simulink model "AdaptiveCruiseControl"  (R2015a)
settings: Solver=ode45  StartTime=0.0  StopTime=250  RelTol=3e-14
libraries: simulink x2
settings Model: CovSFcnEnable=off  Creator=chizom  LastModifiedBy=WORNU CHIZOM

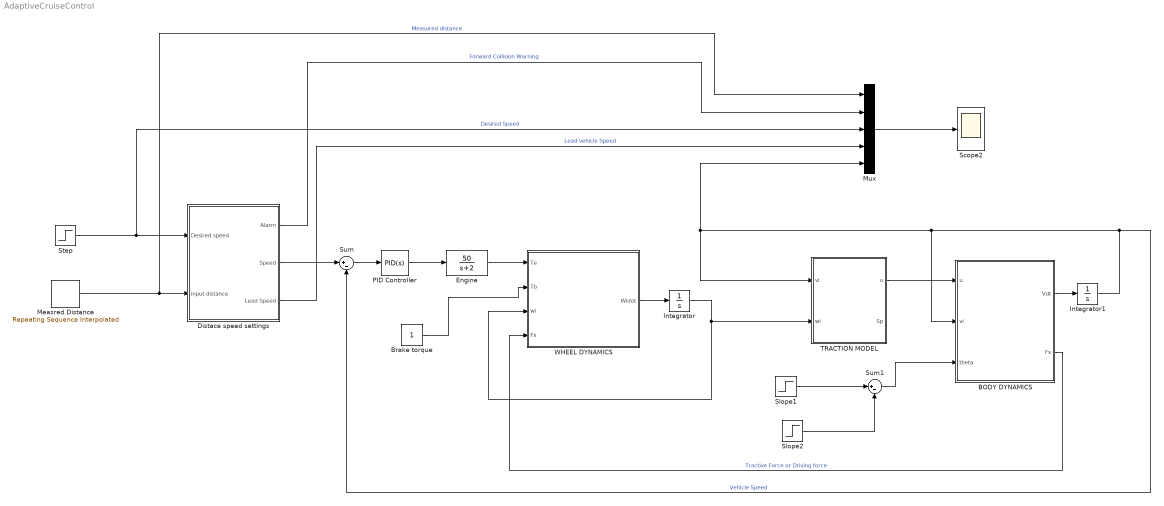
== system AdaptiveCruiseControl ==
  BODY DYNAMICS : Subsystem
  Brake torque : Constant
  Distace speed settings : Subsystem
  Engine : TransferFcn  Numerator=[50]  Denominator=[1 2]
  Integrator : Integrator
  Integrator1 : Integrator  InitialCondition=1
  Measred Distance : simulink/Sources/Repeating Sequence Interpolated  OutValues=[40 30 20 10 8 7 6 6 6 6 6 6].'  TimeValues=[20 40 60 80 100 120 140 160 180 200 220 240].'  LookUpMeth=Interpolation-Use End Values  tsamp=0.001  OutMin=[]  OutMax=[]  OutDataTypeStr=Inherit: Inherit via back propagation  OutDataType=fixdt(0,8)  OutScaling=2^-10
  Mux : Mux  Inputs=5
  PID Controller : simulink/Continuous/PID Controller  Controller=PID  TimeDomain=Continuous-time  SampleTime=-1  IntegratorMethod=Forward Euler  FilterMethod=Forward Euler  Form=Parallel  UseFilter=on  ControllerParametersSource=internal  P=20.88  I=20.88  D=13.92  N=1  InitialConditionSource=internal  InitialConditionForIntegrator=0  InitialConditionForFilter=0  ExternalReset=none  LimitOutput=off  UpperSaturationLimit=inf  LowerSaturationLimit=-inf  LinearizeAsGain=on  AntiWindupMode=none  Kb=1  TrackingMode=off  Kt=1  PParamMin=[]  PParamMax=[]  IParamMin=[]  IParamMax=[]  DParamMin=[]  DParamMax=[]  NParamMin=[]  NParamMax=[]  KbParamMin=[]  KbParamMax=[]  KtParamMin=[]  KtParamMax=[]  POutMin=[]  POutMax=[]  IOutMin=[]  IOutMax=[]  DOutMin=[]  DOutMax=[]  NOutMin=[]  NOutMax=[]  KbOutMin=[]  KbOutMax=[]  KtOutMin=[]  KtOutMax=[]  IntegratorOutMin=[]  IntegratorOutMax=[]  FilterOutMin=[]  FilterOutMax=[]  SumOutMin=[]  SumOutMax=[]  SumI1OutMin=[]  SumI1OutMax=[]  SumI2OutMin=[]  SumI2OutMax=[]  SumI3OutMin=[]  SumI3OutMax=[]  SumDOutMin=[]  SumDOutMax=[]  SaturationOutMin=[]  SaturationOutMax=[]  IntegratorContinuousStateAttributes=''  IntegratorStateMustResolveToSignalObject=off  IntegratorRTWStateStorageClass=Auto  FilterContinuousStateAttributes=''  FilterStateMustResolveToSignalObject=off  FilterRTWStateStorageClass=Auto  DifferentiatorICPrevScaledInput=0  DifferentiatorOutMin=[]  DifferentiatorOutMax=[]
  Scope2 : Scope
      settings: TickLabels=on  ShowLegends=on  TimeRange=250  YMin=0  YMax=70
  Slope1 : Step  Time=100  After=0  SampleTime=0
  Slope2 : Step  Time=200  After=0  SampleTime=0
  Step : Step  Time=0  Before=0.0001  After=30  SampleTime=0
  Sum : Sum  Inputs=|+-
  Sum1 : Sum  Inputs=|+-
  TRACTION MODEL : Subsystem
  WHEEL DYNAMICS : Subsystem
  wires:
  Integrator/1 -> WHEEL DYNAMICS/3(wi), TRACTION MODEL/2(wi)
  WHEEL DYNAMICS/1(Widot) -> Integrator/1
  Engine/1 -> WHEEL DYNAMICS/1(Te)
  TRACTION MODEL/1(u) -> BODY DYNAMICS/1(u)
  BODY DYNAMICS/1(Vdt) -> Integrator1/1
  Integrator1/1 -> TRACTION MODEL/1(vi), Mux/5, BODY DYNAMICS/2(vi), Sum/2  "Vehicle Speed"
  Distace speed settings/2(Speed) -> Sum/1
  Mux/1 -> Scope2/1
  Step/1 -> Mux/3, Distace speed settings/1(Desired speed)  "Desired Speed"
  Measred Distance/1 -> Mux/1, Distace speed settings/2(input distance)  "Measured distance"
  Sum1/1 -> BODY DYNAMICS/3(theta)
  Slope1/1 -> Sum1/1
  Slope2/1 -> Sum1/2
  Sum/1 -> PID Controller/1
  PID Controller/1 -> Engine/1
  Distace speed settings/1(Alarm) -> Mux/2  "Forward Collision Warning"
  Distace speed settings/3(Lead Speed) -> Mux/4  "Lead vehicle Speed"
  BODY DYNAMICS/2(Fx) -> WHEEL DYNAMICS/4(Fx)  "Tractive Force or Driving force"
  Brake torque/1 -> WHEEL DYNAMICS/2(Tb)

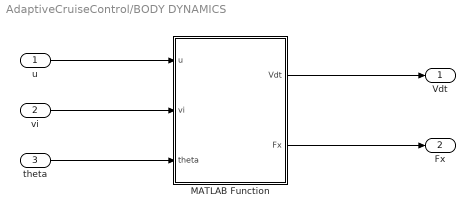
== system AdaptiveCruiseControl/BODY DYNAMICS ==
  u : Inport
  vi : Inport  Port=2
  theta : Inport  Port=3
  MATLAB Function : MATLAB Function  TreatAsAtomicUnit=on
  Vdt : Outport
  Fx : Outport  Port=2
  wires:
  MATLAB Function/1(Vdt) -> Vdt/1
  vi/1 -> MATLAB Function/2(vi)
  theta/1 -> MATLAB Function/3(theta)
  u/1 -> MATLAB Function/1(u)
  MATLAB Function/2(Fx) -> Fx/1

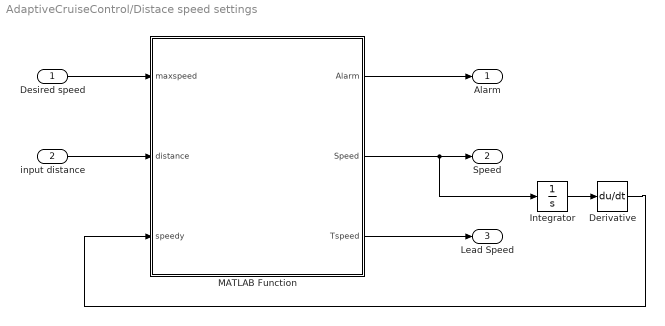
== system AdaptiveCruiseControl/Distace speed settings ==
  Desired speed : Inport
  input distance : Inport  Port=2
  Derivative : Derivative
  Integrator : Integrator
  MATLAB Function : MATLAB Function  TreatAsAtomicUnit=on
  Alarm : Outport
  Speed : Outport  Port=2
  Lead Speed : Outport  Port=3
  wires:
  MATLAB Function/1(Alarm) -> Alarm/1
  Desired speed/1 -> MATLAB Function/1(maxspeed)
  input distance/1 -> MATLAB Function/2(distance)
  MATLAB Function/3(Tspeed) -> Lead Speed/1
  MATLAB Function/2(Speed) -> Integrator/1, Speed/1
  Integrator/1 -> Derivative/1
  Derivative/1 -> MATLAB Function/3(speedy)

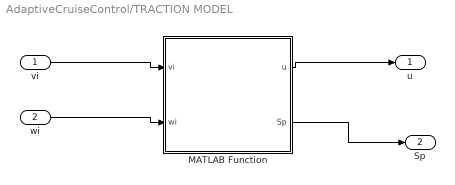
== system AdaptiveCruiseControl/TRACTION MODEL ==
  vi : Inport
  wi : Inport  Port=2
  MATLAB Function : MATLAB Function  TreatAsAtomicUnit=on
  u : Outport
  Sp : Outport  Port=2
  wires:
  vi/1 -> MATLAB Function/1(vi)
  wi/1 -> MATLAB Function/2(wi)
  MATLAB Function/1(u) -> u/1
  MATLAB Function/2(Sp) -> Sp/1

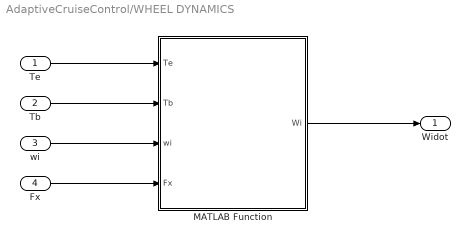
== system AdaptiveCruiseControl/WHEEL DYNAMICS ==
  Te : Inport
  Tb : Inport  Port=2
  wi : Inport  Port=3
  Fx : Inport  Port=4
  MATLAB Function : MATLAB Function  TreatAsAtomicUnit=on
  Widot : Outport
  wires:
  Te/1 -> MATLAB Function/1(Te)
  Tb/1 -> MATLAB Function/2(Tb)
  MATLAB Function/1(Wi) -> Widot/1
  wi/1 -> MATLAB Function/3(wi)
  Fx/1 -> MATLAB Function/4(Fx)

== matlab function AdaptiveCruiseControl/TRACTION MODEL/MATLAB Function ==
  data: u output; vi input; wi input; Sp output
function [u,Sp] = fcn(vi,wi)
% C1, C2, C3 are road condition for dry asphalt

r=0.3; % Radius of wheel
 %Dry Asphalt road%
C1 = 1.2801;
C2 = 23.99;
C3 = 0.52;

Sp = (vi-(r*wi))/vi; %Slip equation
u = C1-C1*exp(-C2*Sp)-C3*Sp; % Equation of friction

== matlab function AdaptiveCruiseControl/WHEEL DYNAMICS/MATLAB Function ==
  data: Te input; Wi output; Tb input; wi input; Fx input
function Wi   = fcn(Te, Tb, wi, Fx)

Jw = 4.5; % Inertia Kg.m^2
r = 0.3; % Radius of Wheel
Cf = 0.1; % Viscous coefficient
Wi = (Te-Tb-wi*Cf-r*Fx)/Jw % Wheel acceleration

== matlab function AdaptiveCruiseControl/BODY DYNAMICS/MATLAB Function ==
  data: u input; Vdt output; vi input; theta input; Fx output
function [Vdt,Fx]  = fcn(u,vi,theta)
%#codegen
M = 1300; % 1500Kg
g = 9.81; % m/s2
Cr = 0.01;				% coefficient of rolling friction
rho = 1.3;				% density of air, kg/m^3
Cd = 0.46;				% drag coefficient
A = 1.6 + 0.00056*(M-765);				% car area, m^2

Fr = M * g * Cr	;		% Rolling friction
Fa = 0.5 * rho * Cd * A * vi*vi;		% Aerodynamic drag
Fg = M * g * sin(theta);		% Road slope force
Fd = Fr + Fa + Fg;			% total deceleration
Fz = M * g * cos(theta); % Normal Force
Fx = 4*u*Fz; % Driving Force

Vdt = (Fx-Fd)/M; % Acceleration of the vehicle

== matlab function AdaptiveCruiseControl/Distace speed settings/MATLAB Function ==
  data: maxspeed input; distance input; Alarm output; Speed output; Tspeed output; speedy input
function [Alarm, Speed,Tspeed] = fcn(maxspeed, distance,speedy)
Alarm1=0;  %Initializing the Alarm
speed1=0;  %Initializing the speed
safe_distance = 5; % Safe distance between both vehicles
THW= 1; %Time Headway
desired_distance = safe_distance + speedy*THW; % Desired Distance
error_distance=distance-desired_distance; % Distance Error
% speedy is the vehicles speed feed back into the system
Tspeed = (speedy + (error_distance*0.1)); % Lead vehicles Speed
min_distance = 2; % Minimum Distance

% Constrain 1
if distance >= desired_distance
    speed1 = maxspeed;
    % Constrain 2
elseif distance <= 3%min_distance
    speed1 = 0;
end
% Constrain 3
if distance <  desired_distance && distance >= min_distance
    if Tspeed>maxspeed
        speed1 = maxspeed;
    else
        speed1 = Tspeed+0.01;
    end
end
%Distance Alert and Forward Collsion Warning
% Constrain 4
if distance <= 40 && distance >20
    Alarm1 = 25; %Distance Alert
    % Constrain 5
elseif distance > min_distance && distance <=20
    Alarm1 = 50; %Forward Collsion Warning
end

Alarm=Alarm1;
Speed=speed1;
